simulink library "NxtrLim"  (R2013b)
settings: Solver=ode45  StartTime=0.0  StopTime=10.0  RelTol=1e-3
libraries: NxtrLim x2
settings Model: Creator=qzwc4r  LastModifiedBy=qzwc4r

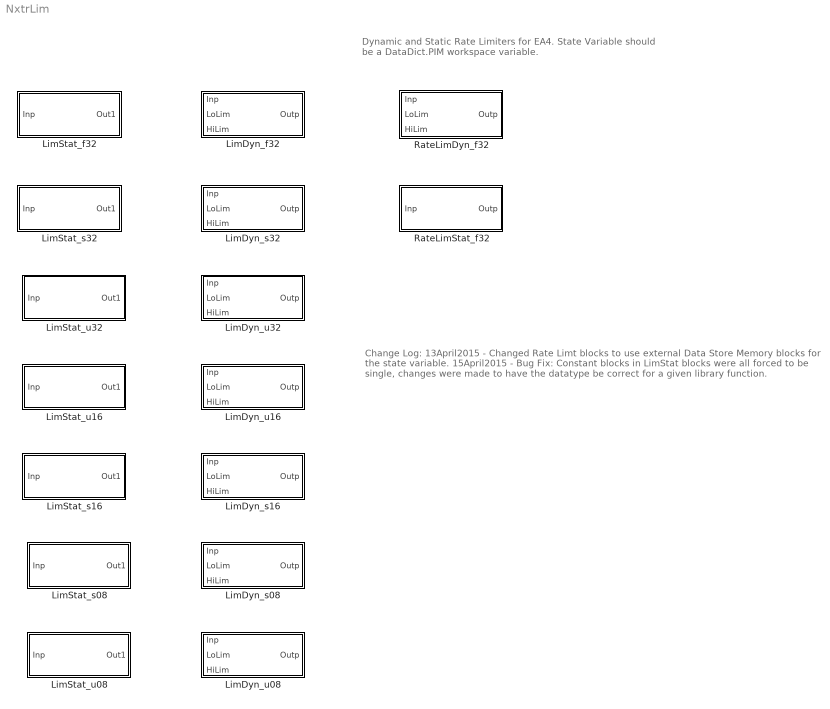
== system NxtrLim ==
  note: Change Log:
      |
      | 13April2015
      | - Changed Rate Limt blocks to use external Data Store Memory blocks for the state variable.
      |
      | 15April2015
      | - Bug Fix: Constant blocks in LimStat blocks were all forced to be single, changes were made
      |    to have the datatype be correct for a given library function.
  note: Dynamic and Static Rate Limiters for EA4.
      | State Variable should be a DataDict.PIM workspace variable.
  LimDyn_f32 : Subsystem  mask(LimDyn_f32){}
      mask Display:
      | Xx = [-0.06, 0.06]*3;
      | Xy = [ 0, 0];
      | Yx = [ 0, 0];
      | Yy = [-0.14, 0.14]*3;
      | 
      | px = [-.06, -0.02, 0.02, 0.06]*3;
      | py = [-.1, -.1, .1, .1]*3;
      | plot(Xx+.5,Xy+.5, Yx+.5,Yy+.5, px+.5,py+.5)
      | 
      | port_label('input',1,'Inp')
      | port_label('input',2,'LoLim')
      | port_label('input',3,'HiLim')
      | port_label('output',1,'Outp')
  LimDyn_s08 : Subsystem  mask(LimDyn_s08){}
      mask Display:
      | Xx = [-0.06, 0.06]*3;
      | Xy = [ 0, 0];
      | Yx = [ 0, 0];
      | Yy = [-0.14, 0.14]*3;
      | 
      | px = [-.06, -0.02, 0.02, 0.06]*3;
      | py = [-.1, -.1, .1, .1]*3;
      | plot(Xx+.5,Xy+.5, Yx+.5,Yy+.5, px+.5,py+.5)
      | 
      | port_label('input',1,'Inp')
      | port_label('input',2,'LoLim')
      | port_label('input',3,'HiLim')
      | port_label('output',1,'Outp')
  LimDyn_s16 : Subsystem  mask(LimDyn_s16){}
      mask Display:
      | Xx = [-0.06, 0.06]*3;
      | Xy = [ 0, 0];
      | Yx = [ 0, 0];
      | Yy = [-0.14, 0.14]*3;
      | 
      | px = [-.06, -0.02, 0.02, 0.06]*3;
      | py = [-.1, -.1, .1, .1]*3;
      | plot(Xx+.5,Xy+.5, Yx+.5,Yy+.5, px+.5,py+.5)
      | 
      | port_label('input',1,'Inp')
      | port_label('input',2,'LoLim')
      | port_label('input',3,'HiLim')
      | port_label('output',1,'Outp')
  LimDyn_s32 : Subsystem  mask(LimDyn_s32){}
      mask Display:
      | Xx = [-0.06, 0.06]*3;
      | Xy = [ 0, 0];
      | Yx = [ 0, 0];
      | Yy = [-0.14, 0.14]*3;
      | 
      | px = [-.06, -0.02, 0.02, 0.06]*3;
      | py = [-.1, -.1, .1, .1]*3;
      | plot(Xx+.5,Xy+.5, Yx+.5,Yy+.5, px+.5,py+.5)
      | 
      | port_label('input',1,'Inp')
      | port_label('input',2,'LoLim')
      | port_label('input',3,'HiLim')
      | port_label('output',1,'Outp')
  LimDyn_u08 : Subsystem  mask(LimDyn_u08){}
      mask Display:
      | Xx = [-0.06, 0.06]*3;
      | Xy = [ 0, 0];
      | Yx = [ 0, 0];
      | Yy = [-0.14, 0.14]*3;
      | 
      | px = [-.06, -0.02, 0.02, 0.06]*3;
      | py = [-.1, -.1, .1, .1]*3;
      | plot(Xx+.5,Xy+.5, Yx+.5,Yy+.5, px+.5,py+.5)
      | 
      | port_label('input',1,'Inp')
      | port_label('input',2,'LoLim')
      | port_label('input',3,'HiLim')
      | port_label('output',1,'Outp')
  LimDyn_u16 : Subsystem  mask(LimDyn_u16){}
      mask Display:
      | Xx = [-0.06, 0.06]*3;
      | Xy = [ 0, 0];
      | Yx = [ 0, 0];
      | Yy = [-0.14, 0.14]*3;
      | 
      | px = [-.06, -0.02, 0.02, 0.06]*3;
      | py = [-.1, -.1, .1, .1]*3;
      | plot(Xx+.5,Xy+.5, Yx+.5,Yy+.5, px+.5,py+.5)
      | 
      | port_label('input',1,'Inp')
      | port_label('input',2,'LoLim')
      | port_label('input',3,'HiLim')
      | port_label('output',1,'Outp')
  LimDyn_u32 : Subsystem  mask(LimDyn_u32){}
      mask Display:
      | Xx = [-0.06, 0.06]*3;
      | Xy = [ 0, 0];
      | Yx = [ 0, 0];
      | Yy = [-0.14, 0.14]*3;
      | 
      | px = [-.06, -0.02, 0.02, 0.06]*3;
      | py = [-.1, -.1, .1, .1]*3;
      | plot(Xx+.5,Xy+.5, Yx+.5,Yy+.5, px+.5,py+.5)
      | 
      | port_label('input',1,'Inp')
      | port_label('input',2,'LoLim')
      | port_label('input',3,'HiLim')
      | port_label('output',1,'Outp')
  LimStat_f32 : Subsystem  mask(LimStat_f32){LoLim=0, HiLim=0}
      mask prompts: LoLim "Lower Limit"; HiLim "Upper Limit"
      settings: AttributesFormatString=|
      | Low Limit: %<LoLim>
      | High Limit:%<HiLim>
      mask Display:
      | Xx = [-0.06, 0.06]*3;
      | Xy = [ 0, 0];
      | Yx = [ 0, 0];
      | Yy = [-0.14, 0.14]*3;
      | 
      | px = [-.06, -0.02, 0.02, 0.06]*3;
      | py = [-.1, -.1, .1, .1]*3;
      | plot(Xx+.5,Xy+.5, Yx+.5,Yy+.5, px+.5,py+.5)
      | 
      | port_label('input',1,'Inp')
      | port_label('output',1,'Outp')
  LimStat_s08 : Subsystem  mask(LimStat_s08){LoLim=0, HiLim=0}
      mask prompts: LoLim "Lower Limit"; HiLim "Upper Limit"
      settings: AttributesFormatString=|
      | Low Limit: %<LoLim>
      | High Limit:%<HiLim>
      mask Display:
      | Xx = [-0.06, 0.06]*3;
      | Xy = [ 0, 0];
      | Yx = [ 0, 0];
      | Yy = [-0.14, 0.14]*3;
      | 
      | px = [-.06, -0.02, 0.02, 0.06]*3;
      | py = [-.1, -.1, .1, .1]*3;
      | plot(Xx+.5,Xy+.5, Yx+.5,Yy+.5, px+.5,py+.5)
      | 
      | port_label('input',1,'Inp')
      | port_label('output',1,'Outp')
  LimStat_s16 : Subsystem  mask(LimStat_s16){LoLim=0, HiLim=0}
      mask prompts: LoLim "Lower Limit"; HiLim "Upper Limit"
      settings: AttributesFormatString=|
      | Low Limit: %<LoLim>
      | High Limit:%<HiLim>
      mask Display:
      | Xx = [-0.06, 0.06]*3;
      | Xy = [ 0, 0];
      | Yx = [ 0, 0];
      | Yy = [-0.14, 0.14]*3;
      | 
      | px = [-.06, -0.02, 0.02, 0.06]*3;
      | py = [-.1, -.1, .1, .1]*3;
      | plot(Xx+.5,Xy+.5, Yx+.5,Yy+.5, px+.5,py+.5)
      | 
      | port_label('input',1,'Inp')
      | port_label('output',1,'Outp')
  LimStat_s32 : Subsystem  mask(LimStat_s32){LoLim=0, HiLim=0}
      mask prompts: LoLim "Lower Limit"; HiLim "Upper Limit"
      settings: AttributesFormatString=|
      | Low Limit: %<LoLim>
      | High Limit:%<HiLim>
      mask Display:
      | Xx = [-0.06, 0.06]*3;
      | Xy = [ 0, 0];
      | Yx = [ 0, 0];
      | Yy = [-0.14, 0.14]*3;
      | 
      | px = [-.06, -0.02, 0.02, 0.06]*3;
      | py = [-.1, -.1, .1, .1]*3;
      | plot(Xx+.5,Xy+.5, Yx+.5,Yy+.5, px+.5,py+.5)
      | 
      | port_label('input',1,'Inp')
      | port_label('output',1,'Outp')
  LimStat_u08 : Subsystem  mask(LimStat_u08){LoLim=0, HiLim=0}
      mask prompts: LoLim "Lower Limit"; HiLim "Upper Limit"
      settings: AttributesFormatString=|
      | Low Limit: %<LoLim>
      | High Limit:%<HiLim>
      mask Display:
      | Xx = [-0.06, 0.06]*3;
      | Xy = [ 0, 0];
      | Yx = [ 0, 0];
      | Yy = [-0.14, 0.14]*3;
      | 
      | px = [-.06, -0.02, 0.02, 0.06]*3;
      | py = [-.1, -.1, .1, .1]*3;
      | plot(Xx+.5,Xy+.5, Yx+.5,Yy+.5, px+.5,py+.5)
      | 
      | port_label('input',1,'Inp')
      | port_label('output',1,'Outp')
  LimStat_u16 : Subsystem  mask(LimStat_u16){LoLim=0, HiLim=0}
      mask prompts: LoLim "Lower Limit"; HiLim "Upper Limit"
      settings: AttributesFormatString=|
      | Low Limit: %<LoLim>
      | High Limit:%<HiLim>
      mask Display:
      | Xx = [-0.06, 0.06]*3;
      | Xy = [ 0, 0];
      | Yx = [ 0, 0];
      | Yy = [-0.14, 0.14]*3;
      | 
      | px = [-.06, -0.02, 0.02, 0.06]*3;
      | py = [-.1, -.1, .1, .1]*3;
      | plot(Xx+.5,Xy+.5, Yx+.5,Yy+.5, px+.5,py+.5)
      | 
      | port_label('input',1,'Inp')
      | port_label('output',1,'Outp')
  LimStat_u32 : Subsystem  mask(LimStat_u32){LoLim=0, HiLim=0}
      mask prompts: LoLim "Lower Limit"; HiLim "Upper Limit"
      settings: AttributesFormatString=|
      | Low Limit: %<LoLim>
      | High Limit:%<HiLim>
      mask Display:
      | Xx = [-0.06, 0.06]*3;
      | Xy = [ 0, 0];
      | Yx = [ 0, 0];
      | Yy = [-0.14, 0.14]*3;
      | 
      | px = [-.06, -0.02, 0.02, 0.06]*3;
      | py = [-.1, -.1, .1, .1]*3;
      | plot(Xx+.5,Xy+.5, Yx+.5,Yy+.5, px+.5,py+.5)
      | 
      | port_label('input',1,'Inp')
      | port_label('output',1,'Outp')
  RateLimDyn_f32 : Subsystem  mask(RateLimDyn_f32){StVar=DefaultValue, Ts=0.002}
      mask prompts: StVar "State Variable"; Ts "Time Step"
      mask init:
      | blk = gcb;
      | set_param([ blk '/Data Store Write'],'DataStoreName',StVar)
      | set_param([ blk '/Data Store Read'],'DataStoreName',StVar)
      settings: AttributesFormatString=StVar: %<StVar>
      mask Display:
      | Xx = [-0.06, 0.06]*3;
      | Xy = [ 0, 0];
      | Yx = [ 0, 0];
      | Yy = [-0.14, 0.14]*3;
      | 
      | px = [-.15, 0.15];
      | py = [-.4, 0.4];
      | plot(Xx+.5,Xy+.5, Yx+.5,Yy+.5, px+.5,py+.5)
      | 
      | port_label('input',1,'Inp')
      | port_label('input',2,'LoLim')
      | port_label('input',3,'HiLim')
      | port_label('output',1,'Outp')
  RateLimStat_f32 : Subsystem  mask(RateLimStat_f32){StVar=DefaultValue, Ts=0.002, LoLim=0, HiLim=0}
      mask prompts: StVar "State Variable"; Ts "Time Step"; LoLim "Lower Limit"; HiLim "Upper Limit"
      mask init:
      | blk = gcb;
      | set_param([ blk '/Data Store Write'],'DataStoreName',StVar)
      | set_param([ blk '/Data Store Read'],'DataStoreName',StVar)
      settings: AttributesFormatString=|
      | StVar: %<StVar>
      | LoLim: %<LoLim>
      | HiLim: %<HiLim>
      mask Display:
      | Xx = [-0.06, 0.06]*3;
      | Xy = [ 0, 0];
      | Yx = [ 0, 0];
      | Yy = [-0.14, 0.14]*3;
      | 
      | px = [-.15, 0.15];
      | py = [-.4, 0.4];
      | plot(Xx+.5,Xy+.5, Yx+.5,Yy+.5, px+.5,py+.5)
      | 
      | port_label('input',1,'Inp')
      | port_label('output',1,'Outp')

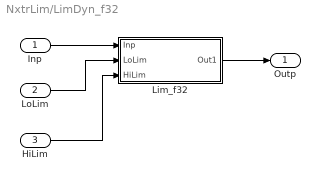
== system NxtrLim/LimDyn_f32 ==
  Inp : Inport
  LoLim : Inport  Port=2
  HiLim : Inport  Port=3
  Lim_f32 : Subsystem
      mask Display:
      | port_label('input',1,'Inp')
      | port_label('input',2,'LoLim')
      | port_label('input',3,'HiLim')
      | port_label('output',1,'Outp')
  Outp : Outport
  wires:
  Lim_f32/1(Out1) -> Outp/1
  Inp/1 -> Lim_f32/1(Inp)
  LoLim/1 -> Lim_f32/2(LoLim)
  HiLim/1 -> Lim_f32/3(HiLim)

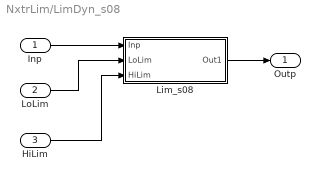
== system NxtrLim/LimDyn_s08 ==
  Inp : Inport
  LoLim : Inport  Port=2
  HiLim : Inport  Port=3
  Lim_s08 : Subsystem
      mask Display:
      | Xx = [-0.06, 0.06]*3;
      | Xy = [ 0, 0];
      | Yx = [ 0, 0];
      | Yy = [-0.14, 0.14]*3;
      | 
      | px = [-.06, -0.02, 0.02, 0.06]*3;
      | py = [-.1, -.1, .1, .1]*3;
      | plot(Xx+.5,Xy+.5, Yx+.5,Yy+.5, px+.5,py+.5)
      | 
      | port_label('input',1,'Inp')
      | port_label('input',2,'LoLim')
      | port_label('input',3,'HiLim')
      | port_label('output',1,'Outp')
  Outp : Outport
  wires:
  HiLim/1 -> Lim_s08/3(HiLim)
  LoLim/1 -> Lim_s08/2(LoLim)
  Inp/1 -> Lim_s08/1(Inp)
  Lim_s08/1(Out1) -> Outp/1

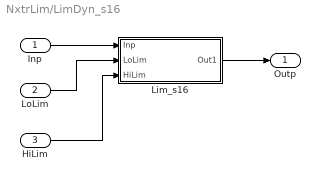
== system NxtrLim/LimDyn_s16 ==
  Inp : Inport
  LoLim : Inport  Port=2
  HiLim : Inport  Port=3
  Lim_s16 : Subsystem
      mask Display:
      | Xx = [-0.06, 0.06]*3;
      | Xy = [ 0, 0];
      | Yx = [ 0, 0];
      | Yy = [-0.14, 0.14]*3;
      | 
      | px = [-.06, -0.02, 0.02, 0.06]*3;
      | py = [-.1, -.1, .1, .1]*3;
      | plot(Xx+.5,Xy+.5, Yx+.5,Yy+.5, px+.5,py+.5)
      | 
      | port_label('input',1,'Inp')
      | port_label('input',2,'LoLim')
      | port_label('input',3,'HiLim')
      | port_label('output',1,'Outp')
  Outp : Outport
  wires:
  Lim_s16/1(Out1) -> Outp/1
  Inp/1 -> Lim_s16/1(Inp)
  LoLim/1 -> Lim_s16/2(LoLim)
  HiLim/1 -> Lim_s16/3(HiLim)

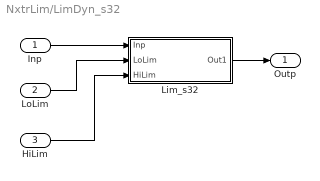
== system NxtrLim/LimDyn_s32 ==
  Inp : Inport
  LoLim : Inport  Port=2
  HiLim : Inport  Port=3
  Lim_s32 : Subsystem
      mask Display:
      | Xx = [-0.06, 0.06]*3;
      | Xy = [ 0, 0];
      | Yx = [ 0, 0];
      | Yy = [-0.14, 0.14]*3;
      | 
      | px = [-.06, -0.02, 0.02, 0.06]*3;
      | py = [-.1, -.1, .1, .1]*3;
      | plot(Xx+.5,Xy+.5, Yx+.5,Yy+.5, px+.5,py+.5)
      | 
      | port_label('input',1,'Inp')
      | port_label('input',2,'LoLim')
      | port_label('input',3,'HiLim')
      | port_label('output',1,'Outp')
  Outp : Outport
  wires:
  HiLim/1 -> Lim_s32/3(HiLim)
  LoLim/1 -> Lim_s32/2(LoLim)
  Inp/1 -> Lim_s32/1(Inp)
  Lim_s32/1(Out1) -> Outp/1

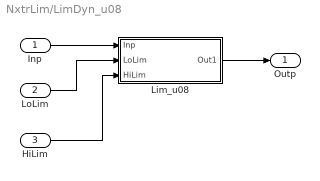
== system NxtrLim/LimDyn_u08 ==
  Inp : Inport
  LoLim : Inport  Port=2
  HiLim : Inport  Port=3
  Lim_u08 : Subsystem
      mask Display:
      | Xx = [-0.06, 0.06]*3;
      | Xy = [ 0, 0];
      | Yx = [ 0, 0];
      | Yy = [-0.14, 0.14]*3;
      | 
      | px = [-.06, -0.02, 0.02, 0.06]*3;
      | py = [-.1, -.1, .1, .1]*3;
      | plot(Xx+.5,Xy+.5, Yx+.5,Yy+.5, px+.5,py+.5)
      | 
      | port_label('input',1,'Inp')
      | port_label('input',2,'LoLim')
      | port_label('input',3,'HiLim')
      | port_label('output',1,'Outp')
  Outp : Outport
  wires:
  Lim_u08/1(Out1) -> Outp/1
  Inp/1 -> Lim_u08/1(Inp)
  LoLim/1 -> Lim_u08/2(LoLim)
  HiLim/1 -> Lim_u08/3(HiLim)

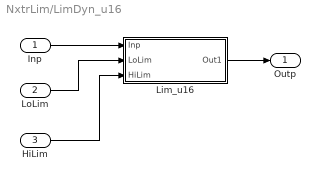
== system NxtrLim/LimDyn_u16 ==
  Inp : Inport
  LoLim : Inport  Port=2
  HiLim : Inport  Port=3
  Lim_u16 : Subsystem
      mask Display:
      | Xx = [-0.06, 0.06]*3;
      | Xy = [ 0, 0];
      | Yx = [ 0, 0];
      | Yy = [-0.14, 0.14]*3;
      | 
      | px = [-.06, -0.02, 0.02, 0.06]*3;
      | py = [-.1, -.1, .1, .1]*3;
      | plot(Xx+.5,Xy+.5, Yx+.5,Yy+.5, px+.5,py+.5)
      | 
      | port_label('input',1,'Inp')
      | port_label('input',2,'LoLim')
      | port_label('input',3,'HiLim')
      | port_label('output',1,'Outp')
  Outp : Outport
  wires:
  HiLim/1 -> Lim_u16/3(HiLim)
  LoLim/1 -> Lim_u16/2(LoLim)
  Inp/1 -> Lim_u16/1(Inp)
  Lim_u16/1(Out1) -> Outp/1

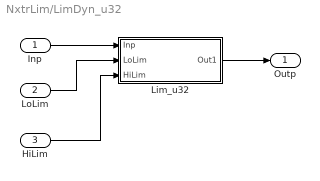
== system NxtrLim/LimDyn_u32 ==
  Inp : Inport
  LoLim : Inport  Port=2
  HiLim : Inport  Port=3
  Lim_u32 : Subsystem
      mask Display:
      | Xx = [-0.06, 0.06]*3;
      | Xy = [ 0, 0];
      | Yx = [ 0, 0];
      | Yy = [-0.14, 0.14]*3;
      | 
      | px = [-.06, -0.02, 0.02, 0.06]*3;
      | py = [-.1, -.1, .1, .1]*3;
      | plot(Xx+.5,Xy+.5, Yx+.5,Yy+.5, px+.5,py+.5)
      | 
      | port_label('input',1,'Inp')
      | port_label('input',2,'LoLim')
      | port_label('input',3,'HiLim')
      | port_label('output',1,'Outp')
  Outp : Outport
  wires:
  Lim_u32/1(Out1) -> Outp/1
  Inp/1 -> Lim_u32/1(Inp)
  LoLim/1 -> Lim_u32/2(LoLim)
  HiLim/1 -> Lim_u32/3(HiLim)

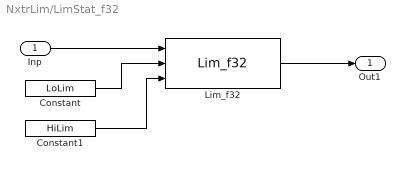
== system NxtrLim/LimStat_f32 ==
  Inp : Inport
  Constant : Constant  Value=LoLim  OutDataTypeStr=single
  Constant1 : Constant  Value=HiLim  OutDataTypeStr=single
  Lim_f32 : S-Function  FunctionName=Lim_f32  EnableBusSupport=off  mask(Legacy Function){SFunctionSpec=single y1 = Lim_f32(single u1, single u2, single u3)}
      mask help:
      | This block allows you to call the legacy functions specified by the following Legacy Code Tool definition:
      | def.SFunctionName = 'Lim_f32';
      | def.OutputFcnSpec = 'single y1 = Lim_f32(single u1, single u2, single u3)';
      | def.HeaderFiles = {'NxtrMath.h', 'Std_Types.h', 'Platform_Types.h', 'Compiler.h', 'Compiler_Cfg.h'};
      | def.IncPaths = {'..\Nexteer_Utilities v3.0.0\SrcFiles'};
      settings: AttributesFormatString=%<Name>
      mask Help: <p>This block was generated automatically by the Legacy Code Tool. For detailed help on this tool, call<a href="matlab:legacy_code('help')"> legacy_code('help')</a>.</p>
      mask Display:
      | port_label('input',1,'Inp')
      | port_label('input',2,'LoLim')
      | port_label('input',3,'HiLim')
      | port_label('output',1,'Outp')
  Out1 : Outport
  wires:
  Lim_f32/1 -> Out1/1
  Constant1/1 -> Lim_f32/3
  Constant/1 -> Lim_f32/2
  Inp/1 -> Lim_f32/1

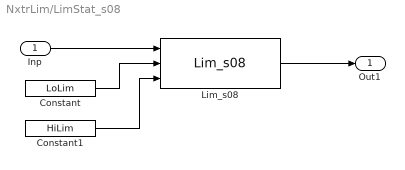
== system NxtrLim/LimStat_s08 ==
  Inp : Inport
  Constant : Constant  Value=LoLim  OutDataTypeStr=int8
  Constant1 : Constant  Value=HiLim  OutDataTypeStr=int8
  Lim_s08 : S-Function  FunctionName=Lim_s08  EnableBusSupport=off  mask(Legacy Function){SFunctionSpec=int8 y1 = Lim_s08(  int8 u1,   int8 u2,   int8 u3), ShowSpec=on}
      mask prompts: ShowSpec "Display function specification"
      mask help:
      | This block allows you to call the legacy functions specified by the following Legacy Code Tool definition:
      | def.SFunctionName = 'Lim_s08';
      | def.OutputFcnSpec = '  int8 y1 = Lim_s08(  int8 u1,   int8 u2,   int8 u3)';
      | def.HeaderFiles = {'NxtrMath.h', 'Std_Types.h', 'Platform_Types.h', 'Compiler.h', 'Compiler_Cfg.h'};
      | def.IncPaths = {'..\Nexteer_Utilities v3.0.0\SrcFiles'};
      settings: AttributesFormatString=%<Name>
      mask Help: <p>This block was generated automatically by the Legacy Code Tool. For detailed help on this tool, call<a href="matlab:legacy_code('help')"> legacy_code('help')</a>.</p>
      mask Callback ShowSpec:
      | if strcmp(get_param(gcbh, 'ShowSpec'), 'on')
      |   set_param(gcbh, 'MaskDisplay', sprintf('fprintf(''%s'');', get_param(gcbh, 'SFunctionSpec')));
      | else
      |   set_param(gcbh, 'MaskDisplay', sprintf('fprintf(''%s'');', get_param(gcbh, 'FunctionName')));
      | end
      mask Display:
      | Xx = [-0.06, 0.06]*3;
      | Xy = [ 0, 0];
      | Yx = [ 0, 0];
      | Yy = [-0.14, 0.14]*3;
      | 
      | px = [-.06, -0.02, 0.02, 0.06]*3;
      | py = [-.1, -.1, .1, .1]*3;
      | plot(Xx+.5,Xy+.5, Yx+.5,Yy+.5, px+.5,py+.5)
      | port_label('input',1,'Inp')
      | port_label('input',2,'LoLim')
      | port_label('input',3,'HiLim')
      | port_label('output',1,'Outp')
  Out1 : Outport
  wires:
  Inp/1 -> Lim_s08/1
  Constant/1 -> Lim_s08/2
  Constant1/1 -> Lim_s08/3
  Lim_s08/1 -> Out1/1

== system NxtrLim/LimStat_s16 ==
  Inp : Inport
  Constant : Constant  Value=LoLim  OutDataTypeStr=int16
  Constant1 : Constant  Value=HiLim  OutDataTypeStr=int16
  Lim_s16 : S-Function  FunctionName=Lim_s16  EnableBusSupport=off  mask(Legacy Function){SFunctionSpec=int16 y1 = Lim_s16( int16 u1,  int16 u2,  int16 u3)}
      mask help:
      | This block allows you to call the legacy functions specified by the following Legacy Code Tool definition:
      | def.SFunctionName = 'Lim_s16';
      | def.OutputFcnSpec = ' int16 y1 = Lim_s16( int16 u1,  int16 u2,  int16 u3)';
      | def.HeaderFiles = {'NxtrMath.h', 'Std_Types.h', 'Platform_Types.h', 'Compiler.h', 'Compiler_Cfg.h'};
      | def.IncPaths = {'..\Nexteer_Utilities v3.0.0\SrcFiles'};
      settings: AttributesFormatString=%<Name>
      mask Help: <p>This block was generated automatically by the Legacy Code Tool. For detailed help on this tool, call<a href="matlab:legacy_code('help')"> legacy_code('help')</a>.</p>
      mask Display:
      | Xx = [-0.06, 0.06]*3;
      | Xy = [ 0, 0];
      | Yx = [ 0, 0];
      | Yy = [-0.14, 0.14]*3;
      | 
      | px = [-.06, -0.02, 0.02, 0.06]*3;
      | py = [-.1, -.1, .1, .1]*3;
      | plot(Xx+.5,Xy+.5, Yx+.5,Yy+.5, px+.5,py+.5)
      | port_label('input',1,'Inp')
      | port_label('input',2,'LoLim')
      | port_label('input',3,'HiLim')
      | port_label('output',1,'Outp')
  Out1 : Outport
  wires:
  Lim_s16/1 -> Out1/1
  Constant1/1 -> Lim_s16/3
  Constant/1 -> Lim_s16/2
  Inp/1 -> Lim_s16/1

== system NxtrLim/LimStat_s32 ==
  Inp : Inport
  Constant : Constant  Value=LoLim  OutDataTypeStr=int32
  Constant1 : Constant  Value=HiLim  OutDataTypeStr=int32
  Lim_s32 : Subsystem
      mask Display:
      | Xx = [-0.06, 0.06]*3;
      | Xy = [ 0, 0];
      | Yx = [ 0, 0];
      | Yy = [-0.14, 0.14]*3;
      | 
      | px = [-.06, -0.02, 0.02, 0.06]*3;
      | py = [-.1, -.1, .1, .1]*3;
      | plot(Xx+.5,Xy+.5, Yx+.5,Yy+.5, px+.5,py+.5)
      | 
      | port_label('input',1,'Inp')
      | port_label('input',2,'LoLim')
      | port_label('input',3,'HiLim')
      | port_label('output',1,'Outp')
  Out1 : Outport
  wires:
  Inp/1 -> Lim_s32/1(Inp)
  Constant/1 -> Lim_s32/2(LoLim)
  Constant1/1 -> Lim_s32/3(HiLim)
  Lim_s32/1(Out1) -> Out1/1

== system NxtrLim/LimStat_u08 ==
  Inp : Inport
  Constant : Constant  Value=LoLim  OutDataTypeStr=uint8
  Constant1 : Constant  Value=HiLim  OutDataTypeStr=uint8
  Lim_u08 : S-Function  FunctionName=Lim_u08  EnableBusSupport=off  mask(Legacy Function){SFunctionSpec=uint8 y1 = Lim_u08( uint8 u1,  uint8 u2,  uint8 u3), ShowSpec=on}
      mask prompts: ShowSpec "Display function specification"
      mask help:
      | This block allows you to call the legacy functions specified by the following Legacy Code Tool definition:
      | def.SFunctionName = 'Lim_u08';
      | def.OutputFcnSpec = ' uint8 y1 = Lim_u08( uint8 u1,  uint8 u2,  uint8 u3)';
      | def.HeaderFiles = {'NxtrMath.h', 'Std_Types.h', 'Platform_Types.h', 'Compiler.h', 'Compiler_Cfg.h'};
      | def.IncPaths = {'..\Nexteer_Utilities v3.0.0\SrcFiles'};
      settings: AttributesFormatString=%<Name>
      mask Help: <p>This block was generated automatically by the Legacy Code Tool. For detailed help on this tool, call<a href="matlab:legacy_code('help')"> legacy_code('help')</a>.</p>
      mask Callback ShowSpec:
      | if strcmp(get_param(gcbh, 'ShowSpec'), 'on')
      |   set_param(gcbh, 'MaskDisplay', sprintf('fprintf(''%s'');', get_param(gcbh, 'SFunctionSpec')));
      | else
      |   set_param(gcbh, 'MaskDisplay', sprintf('fprintf(''%s'');', get_param(gcbh, 'FunctionName')));
      | end
      mask Display:
      | Xx = [-0.06, 0.06]*3;
      | Xy = [ 0, 0];
      | Yx = [ 0, 0];
      | Yy = [-0.14, 0.14]*3;
      | 
      | px = [-.06, -0.02, 0.02, 0.06]*3;
      | py = [-.1, -.1, .1, .1]*3;
      | plot(Xx+.5,Xy+.5, Yx+.5,Yy+.5, px+.5,py+.5)
      | port_label('input',1,'Inp')
      | port_label('input',2,'LoLim')
      | port_label('input',3,'HiLim')
      | port_label('output',1,'Outp')
  Out1 : Outport
  wires:
  Lim_u08/1 -> Out1/1
  Constant1/1 -> Lim_u08/3
  Constant/1 -> Lim_u08/2
  Inp/1 -> Lim_u08/1

== system NxtrLim/LimStat_u16 ==
  Inp : Inport
  Constant : Constant  Value=LoLim  OutDataTypeStr=uint16
  Constant1 : Constant  Value=HiLim  OutDataTypeStr=uint16
  Lim_u16 : S-Function  FunctionName=Lim_u16  EnableBusSupport=off  mask(Legacy Function){SFunctionSpec=uint16 y1 = Lim_u16(uint16 u1, uint16 u2, uint16 u3)}
      mask help:
      | This block allows you to call the legacy functions specified by the following Legacy Code Tool definition:
      | def.SFunctionName = 'Lim_u16';
      | def.OutputFcnSpec = 'uint16 y1 = Lim_u16(uint16 u1, uint16 u2, uint16 u3)';
      | def.HeaderFiles = {'NxtrMath.h', 'Std_Types.h', 'Platform_Types.h', 'Compiler.h', 'Compiler_Cfg.h'};
      | def.IncPaths = {'..\Nexteer_Utilities v3.0.0\SrcFiles'};
      settings: AttributesFormatString=%<Name>
      mask Help: <p>This block was generated automatically by the Legacy Code Tool. For detailed help on this tool, call<a href="matlab:legacy_code('help')"> legacy_code('help')</a>.</p>
      mask Display:
      | Xx = [-0.06, 0.06]*3;
      | Xy = [ 0, 0];
      | Yx = [ 0, 0];
      | Yy = [-0.14, 0.14]*3;
      | 
      | px = [-.06, -0.02, 0.02, 0.06]*3;
      | py = [-.1, -.1, .1, .1]*3;
      | plot(Xx+.5,Xy+.5, Yx+.5,Yy+.5, px+.5,py+.5)
      | port_label('input',1,'Inp')
      | port_label('input',2,'LoLim')
      | port_label('input',3,'HiLim')
      | port_label('output',1,'Outp')
  Out1 : Outport
  wires:
  Inp/1 -> Lim_u16/1
  Constant/1 -> Lim_u16/2
  Constant1/1 -> Lim_u16/3
  Lim_u16/1 -> Out1/1

== system NxtrLim/LimStat_u32 ==
  Inp : Inport
  Constant : Constant  Value=LoLim  OutDataTypeStr=uint32
  Constant1 : Constant  Value=HiLim  OutDataTypeStr=uint32
  Lim_u32 : S-Function  FunctionName=Lim_u32  EnableBusSupport=off  mask(Legacy Function){SFunctionSpec=uint32 y1 = Lim_u32(uint32 u1, uint32 u2, uint32 u3)}
      mask help:
      | This block allows you to call the legacy functions specified by the following Legacy Code Tool definition:
      | def.SFunctionName = 'Lim_u32';
      | def.OutputFcnSpec = 'uint32 y1 = Lim_u32(uint32 u1, uint32 u2, uint32 u3)';
      | def.HeaderFiles = {'NxtrMath.h', 'Std_Types.h', 'Platform_Types.h', 'Compiler.h', 'Compiler_Cfg.h'};
      | def.IncPaths = {'..\Nexteer_Utilities v3.0.0\SrcFiles'};
      settings: AttributesFormatString=%<Name>
      mask Help: <p>This block was generated automatically by the Legacy Code Tool. For detailed help on this tool, call<a href="matlab:legacy_code('help')"> legacy_code('help')</a>.</p>
      mask Display:
      | Xx = [-0.06, 0.06]*3;
      | Xy = [ 0, 0];
      | Yx = [ 0, 0];
      | Yy = [-0.14, 0.14]*3;
      | 
      | px = [-.06, -0.02, 0.02, 0.06]*3;
      | py = [-.1, -.1, .1, .1]*3;
      | plot(Xx+.5,Xy+.5, Yx+.5,Yy+.5, px+.5,py+.5)
      | port_label('input',1,'Inp')
      | port_label('input',2,'LoLim')
      | port_label('input',3,'HiLim')
      | port_label('output',1,'Outp')
  Out1 : Outport
  wires:
  Lim_u32/1 -> Out1/1
  Constant1/1 -> Lim_u32/3
  Constant/1 -> Lim_u32/2
  Inp/1 -> Lim_u32/1

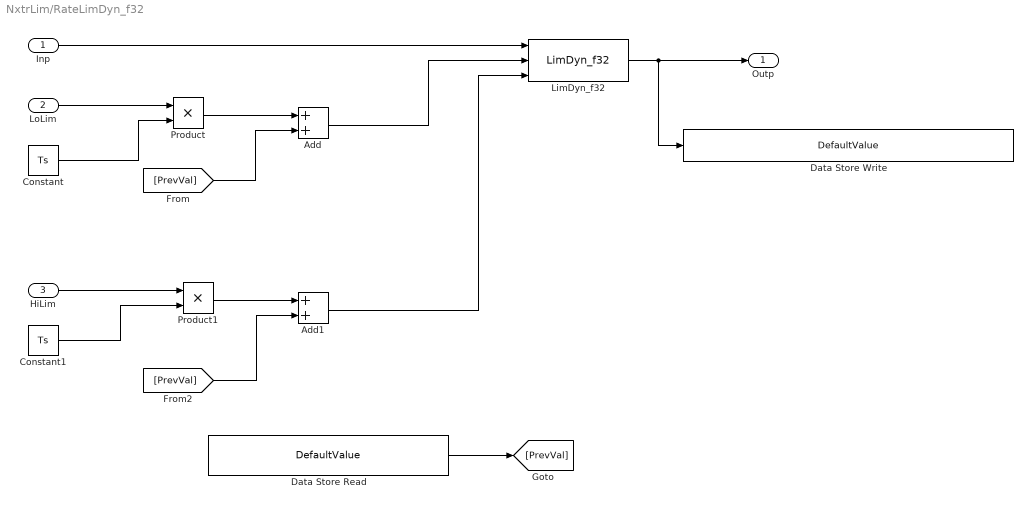
== system NxtrLim/RateLimDyn_f32 ==
  Inp : Inport
  LoLim : Inport  Port=2
  HiLim : Inport  Port=3
  Add : Sum
  Add1 : Sum
  Constant : Constant  Value=Ts
  Constant1 : Constant  Value=Ts
  Data Store Read : DataStoreRead  DataStoreName=DefaultValue
  Data Store Write : DataStoreWrite  DataStoreName=DefaultValue
  LimDyn_f32 : NxtrLim/LimDyn_f32
  Product : Product
  Product1 : Product
  Outp : Outport
  wires:
  Inp/1 -> LimDyn_f32/1
  LimDyn_f32/1 -> Data Store Write/1, Outp/1
  Data Store Read/1 -> [PrevVal]
  LoLim/1 -> Product/1
  Constant/1 -> Product/2
  Product/1 -> Add/1
  HiLim/1 -> Product1/1
  Constant1/1 -> Product1/2
  Product1/1 -> Add1/1
  Add/1 -> LimDyn_f32/2
  Add1/1 -> LimDyn_f32/3
  [PrevVal] -> Add/2
  [PrevVal] -> Add1/2

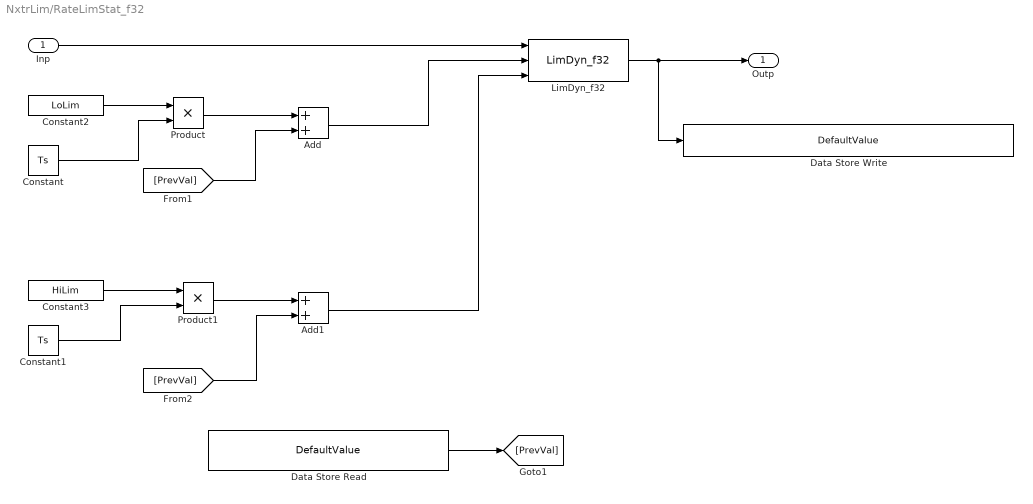
== system NxtrLim/RateLimStat_f32 ==
  Inp : Inport
  Add : Sum
  Add1 : Sum
  Constant : Constant  Value=Ts
  Constant1 : Constant  Value=Ts
  Constant2 : Constant  Value=LoLim
  Constant3 : Constant  Value=HiLim
  Data Store Read : DataStoreRead  DataStoreName=DefaultValue
  Data Store Write : DataStoreWrite  DataStoreName=DefaultValue
  LimDyn_f32 : NxtrLim/LimDyn_f32
  Product : Product
  Product1 : Product
  Outp : Outport
  wires:
  [PrevVal] -> Add1/2
  [PrevVal] -> Add/2
  Add1/1 -> LimDyn_f32/3
  Add/1 -> LimDyn_f32/2
  Product1/1 -> Add1/1
  Constant1/1 -> Product1/2
  Constant3/1 -> Product1/1
  Product/1 -> Add/1
  Constant/1 -> Product/2
  Constant2/1 -> Product/1
  Data Store Read/1 -> [PrevVal]
  LimDyn_f32/1 -> Data Store Write/1, Outp/1
  Inp/1 -> LimDyn_f32/1

== system NxtrLim/LimDyn_f32/Lim_f32 ==
  Inp : Inport
  LoLim : Inport  Port=2
  HiLim : Inport  Port=3
  Lim_f32 : S-Function  FunctionName=Lim_f32  EnableBusSupport=off  mask(Legacy Function){SFunctionSpec=single y1 = Lim_f32(single u1, single u2, single u3)}
      mask help:
      | This block allows you to call the legacy functions specified by the following Legacy Code Tool definition:
      | def.SFunctionName = 'Lim_f32';
      | def.OutputFcnSpec = 'single y1 = Lim_f32(single u1, single u2, single u3)';
      | def.HeaderFiles = {'NxtrMath.h', 'Std_Types.h', 'Platform_Types.h', 'Compiler.h', 'Compiler_Cfg.h'};
      | def.IncPaths = {'..\Nexteer_Utilities v3.0.0\SrcFiles'};
      settings: AttributesFormatString=%<Name>
      mask Help: <p>This block was generated automatically by the Legacy Code Tool. For detailed help on this tool, call<a href="matlab:legacy_code('help')"> legacy_code('help')</a>.</p>
      mask Display:
      | port_label('input',1,'Inp')
      | port_label('input',2,'LoLim')
      | port_label('input',3,'HiLim')
      | port_label('output',1,'Outp')
  Out1 : Outport
  wires:
  Lim_f32/1 -> Out1/1
  HiLim/1 -> Lim_f32/3
  LoLim/1 -> Lim_f32/2
  Inp/1 -> Lim_f32/1

== system NxtrLim/LimDyn_s08/Lim_s08 ==
  Inp : Inport
  LoLim : Inport  Port=2
  HiLim : Inport  Port=3
  Lim_s08 : S-Function  FunctionName=Lim_s08  EnableBusSupport=off  mask(Legacy Function){SFunctionSpec=int8 y1 = Lim_s08(  int8 u1,   int8 u2,   int8 u3), ShowSpec=on}
      mask prompts: ShowSpec "Display function specification"
      mask help:
      | This block allows you to call the legacy functions specified by the following Legacy Code Tool definition:
      | def.SFunctionName = 'Lim_s08';
      | def.OutputFcnSpec = '  int8 y1 = Lim_s08(  int8 u1,   int8 u2,   int8 u3)';
      | def.HeaderFiles = {'NxtrMath.h', 'Std_Types.h', 'Platform_Types.h', 'Compiler.h', 'Compiler_Cfg.h'};
      | def.IncPaths = {'..\Nexteer_Utilities v3.0.0\SrcFiles'};
      settings: AttributesFormatString=%<Name>
      mask Help: <p>This block was generated automatically by the Legacy Code Tool. For detailed help on this tool, call<a href="matlab:legacy_code('help')"> legacy_code('help')</a>.</p>
      mask Callback ShowSpec:
      | if strcmp(get_param(gcbh, 'ShowSpec'), 'on')
      |   set_param(gcbh, 'MaskDisplay', sprintf('fprintf(''%s'');', get_param(gcbh, 'SFunctionSpec')));
      | else
      |   set_param(gcbh, 'MaskDisplay', sprintf('fprintf(''%s'');', get_param(gcbh, 'FunctionName')));
      | end
      mask Display:
      | Xx = [-0.06, 0.06]*3;
      | Xy = [ 0, 0];
      | Yx = [ 0, 0];
      | Yy = [-0.14, 0.14]*3;
      | 
      | px = [-.06, -0.02, 0.02, 0.06]*3;
      | py = [-.1, -.1, .1, .1]*3;
      | plot(Xx+.5,Xy+.5, Yx+.5,Yy+.5, px+.5,py+.5)
      | port_label('input',1,'Inp')
      | port_label('input',2,'LoLim')
      | port_label('input',3,'HiLim')
      | port_label('output',1,'Outp')
  Out1 : Outport
  wires:
  Inp/1 -> Lim_s08/1
  LoLim/1 -> Lim_s08/2
  HiLim/1 -> Lim_s08/3
  Lim_s08/1 -> Out1/1

== system NxtrLim/LimDyn_s16/Lim_s16 ==
  Inp : Inport
  LoLim : Inport  Port=2
  HiLim : Inport  Port=3
  Lim_s16 : S-Function  FunctionName=Lim_s16  EnableBusSupport=off  mask(Legacy Function){SFunctionSpec=int16 y1 = Lim_s16( int16 u1,  int16 u2,  int16 u3)}
      mask help:
      | This block allows you to call the legacy functions specified by the following Legacy Code Tool definition:
      | def.SFunctionName = 'Lim_s16';
      | def.OutputFcnSpec = ' int16 y1 = Lim_s16( int16 u1,  int16 u2,  int16 u3)';
      | def.HeaderFiles = {'NxtrMath.h', 'Std_Types.h', 'Platform_Types.h', 'Compiler.h', 'Compiler_Cfg.h'};
      | def.IncPaths = {'..\Nexteer_Utilities v3.0.0\SrcFiles'};
      settings: AttributesFormatString=%<Name>
      mask Help: <p>This block was generated automatically by the Legacy Code Tool. For detailed help on this tool, call<a href="matlab:legacy_code('help')"> legacy_code('help')</a>.</p>
      mask Display:
      | Xx = [-0.06, 0.06]*3;
      | Xy = [ 0, 0];
      | Yx = [ 0, 0];
      | Yy = [-0.14, 0.14]*3;
      | 
      | px = [-.06, -0.02, 0.02, 0.06]*3;
      | py = [-.1, -.1, .1, .1]*3;
      | plot(Xx+.5,Xy+.5, Yx+.5,Yy+.5, px+.5,py+.5)
      | port_label('input',1,'Inp')
      | port_label('input',2,'LoLim')
      | port_label('input',3,'HiLim')
      | port_label('output',1,'Outp')
  Out1 : Outport
  wires:
  Lim_s16/1 -> Out1/1
  HiLim/1 -> Lim_s16/3
  LoLim/1 -> Lim_s16/2
  Inp/1 -> Lim_s16/1

== system NxtrLim/LimDyn_s32/Lim_s32 ==
  Inp : Inport
  LoLim : Inport  Port=2
  HiLim : Inport  Port=3
  Lim_s32 : S-Function  FunctionName=Lim_s32  EnableBusSupport=off  mask(Legacy Function){SFunctionSpec=int32 y1 = Lim_s32( int32 u1,  int32 u2,  int32 u3)}
      mask help:
      | This block allows you to call the legacy functions specified by the following Legacy Code Tool definition:
      | def.SFunctionName = 'Lim_s32';
      | def.OutputFcnSpec = ' int32 y1 = Lim_s32( int32 u1,  int32 u2,  int32 u3)';
      | def.HeaderFiles = {'NxtrMath.h', 'Std_Types.h', 'Platform_Types.h', 'Compiler.h', 'Compiler_Cfg.h'};
      | def.IncPaths = {'..\Nexteer_Utilities v3.0.0\SrcFiles'};
      settings: AttributesFormatString=%<Name>
      mask Help: <p>This block was generated automatically by the Legacy Code Tool. For detailed help on this tool, call<a href="matlab:legacy_code('help')"> legacy_code('help')</a>.</p>
      mask Display:
      | Xx = [-0.06, 0.06]*3;
      | Xy = [ 0, 0];
      | Yx = [ 0, 0];
      | Yy = [-0.14, 0.14]*3;
      | 
      | px = [-.06, -0.02, 0.02, 0.06]*3;
      | py = [-.1, -.1, .1, .1]*3;
      | plot(Xx+.5,Xy+.5, Yx+.5,Yy+.5, px+.5,py+.5)
      | port_label('input',1,'Inp')
      | port_label('input',2,'LoLim')
      | port_label('input',3,'HiLim')
      | port_label('output',1,'Outp')
  Out1 : Outport
  wires:
  Inp/1 -> Lim_s32/1
  LoLim/1 -> Lim_s32/2
  HiLim/1 -> Lim_s32/3
  Lim_s32/1 -> Out1/1

== system NxtrLim/LimDyn_u08/Lim_u08 ==
  Inp : Inport
  LoLim : Inport  Port=2
  HiLim : Inport  Port=3
  Lim_u08 : S-Function  FunctionName=Lim_u08  EnableBusSupport=off  mask(Legacy Function){SFunctionSpec=uint8 y1 = Lim_u08( uint8 u1,  uint8 u2,  uint8 u3), ShowSpec=on}
      mask prompts: ShowSpec "Display function specification"
      mask help:
      | This block allows you to call the legacy functions specified by the following Legacy Code Tool definition:
      | def.SFunctionName = 'Lim_u08';
      | def.OutputFcnSpec = ' uint8 y1 = Lim_u08( uint8 u1,  uint8 u2,  uint8 u3)';
      | def.HeaderFiles = {'NxtrMath.h', 'Std_Types.h', 'Platform_Types.h', 'Compiler.h', 'Compiler_Cfg.h'};
      | def.IncPaths = {'..\Nexteer_Utilities v3.0.0\SrcFiles'};
      settings: AttributesFormatString=%<Name>
      mask Help: <p>This block was generated automatically by the Legacy Code Tool. For detailed help on this tool, call<a href="matlab:legacy_code('help')"> legacy_code('help')</a>.</p>
      mask Callback ShowSpec:
      | if strcmp(get_param(gcbh, 'ShowSpec'), 'on')
      |   set_param(gcbh, 'MaskDisplay', sprintf('fprintf(''%s'');', get_param(gcbh, 'SFunctionSpec')));
      | else
      |   set_param(gcbh, 'MaskDisplay', sprintf('fprintf(''%s'');', get_param(gcbh, 'FunctionName')));
      | end
      mask Display:
      | Xx = [-0.06, 0.06]*3;
      | Xy = [ 0, 0];
      | Yx = [ 0, 0];
      | Yy = [-0.14, 0.14]*3;
      | 
      | px = [-.06, -0.02, 0.02, 0.06]*3;
      | py = [-.1, -.1, .1, .1]*3;
      | plot(Xx+.5,Xy+.5, Yx+.5,Yy+.5, px+.5,py+.5)
      | port_label('input',1,'Inp')
      | port_label('input',2,'LoLim')
      | port_label('input',3,'HiLim')
      | port_label('output',1,'Outp')
  Out1 : Outport
  wires:
  Lim_u08/1 -> Out1/1
  HiLim/1 -> Lim_u08/3
  LoLim/1 -> Lim_u08/2
  Inp/1 -> Lim_u08/1

== system NxtrLim/LimDyn_u16/Lim_u16 ==
  Inp : Inport
  LoLim : Inport  Port=2
  HiLim : Inport  Port=3
  Lim_u16 : S-Function  FunctionName=Lim_u16  EnableBusSupport=off  mask(Legacy Function){SFunctionSpec=uint16 y1 = Lim_u16(uint16 u1, uint16 u2, uint16 u3)}
      mask help:
      | This block allows you to call the legacy functions specified by the following Legacy Code Tool definition:
      | def.SFunctionName = 'Lim_u16';
      | def.OutputFcnSpec = 'uint16 y1 = Lim_u16(uint16 u1, uint16 u2, uint16 u3)';
      | def.HeaderFiles = {'NxtrMath.h', 'Std_Types.h', 'Platform_Types.h', 'Compiler.h', 'Compiler_Cfg.h'};
      | def.IncPaths = {'..\Nexteer_Utilities v3.0.0\SrcFiles'};
      settings: AttributesFormatString=%<Name>
      mask Help: <p>This block was generated automatically by the Legacy Code Tool. For detailed help on this tool, call<a href="matlab:legacy_code('help')"> legacy_code('help')</a>.</p>
      mask Display:
      | Xx = [-0.06, 0.06]*3;
      | Xy = [ 0, 0];
      | Yx = [ 0, 0];
      | Yy = [-0.14, 0.14]*3;
      | 
      | px = [-.06, -0.02, 0.02, 0.06]*3;
      | py = [-.1, -.1, .1, .1]*3;
      | plot(Xx+.5,Xy+.5, Yx+.5,Yy+.5, px+.5,py+.5)
      | port_label('input',1,'Inp')
      | port_label('input',2,'LoLim')
      | port_label('input',3,'HiLim')
      | port_label('output',1,'Outp')
  Out1 : Outport
  wires:
  Inp/1 -> Lim_u16/1
  LoLim/1 -> Lim_u16/2
  HiLim/1 -> Lim_u16/3
  Lim_u16/1 -> Out1/1

== system NxtrLim/LimDyn_u32/Lim_u32 ==
  Inp : Inport
  LoLim : Inport  Port=2
  HiLim : Inport  Port=3
  Lim_u32 : S-Function  FunctionName=Lim_u32  EnableBusSupport=off  mask(Legacy Function){SFunctionSpec=uint32 y1 = Lim_u32(uint32 u1, uint32 u2, uint32 u3)}
      mask help:
      | This block allows you to call the legacy functions specified by the following Legacy Code Tool definition:
      | def.SFunctionName = 'Lim_u32';
      | def.OutputFcnSpec = 'uint32 y1 = Lim_u32(uint32 u1, uint32 u2, uint32 u3)';
      | def.HeaderFiles = {'NxtrMath.h', 'Std_Types.h', 'Platform_Types.h', 'Compiler.h', 'Compiler_Cfg.h'};
      | def.IncPaths = {'..\Nexteer_Utilities v3.0.0\SrcFiles'};
      settings: AttributesFormatString=%<Name>
      mask Help: <p>This block was generated automatically by the Legacy Code Tool. For detailed help on this tool, call<a href="matlab:legacy_code('help')"> legacy_code('help')</a>.</p>
      mask Display:
      | Xx = [-0.06, 0.06]*3;
      | Xy = [ 0, 0];
      | Yx = [ 0, 0];
      | Yy = [-0.14, 0.14]*3;
      | 
      | px = [-.06, -0.02, 0.02, 0.06]*3;
      | py = [-.1, -.1, .1, .1]*3;
      | plot(Xx+.5,Xy+.5, Yx+.5,Yy+.5, px+.5,py+.5)
      | port_label('input',1,'Inp')
      | port_label('input',2,'LoLim')
      | port_label('input',3,'HiLim')
      | port_label('output',1,'Outp')
  Out1 : Outport
  wires:
  Lim_u32/1 -> Out1/1
  HiLim/1 -> Lim_u32/3
  LoLim/1 -> Lim_u32/2
  Inp/1 -> Lim_u32/1

== system NxtrLim/LimStat_s32/Lim_s32 ==
  Inp : Inport
  LoLim : Inport  Port=2
  HiLim : Inport  Port=3
  Lim_s32 : S-Function  FunctionName=Lim_s32  EnableBusSupport=off  mask(Legacy Function){SFunctionSpec=int32 y1 = Lim_s32( int32 u1,  int32 u2,  int32 u3)}
      mask help:
      | This block allows you to call the legacy functions specified by the following Legacy Code Tool definition:
      | def.SFunctionName = 'Lim_s32';
      | def.OutputFcnSpec = ' int32 y1 = Lim_s32( int32 u1,  int32 u2,  int32 u3)';
      | def.HeaderFiles = {'NxtrMath.h', 'Std_Types.h', 'Platform_Types.h', 'Compiler.h', 'Compiler_Cfg.h'};
      | def.IncPaths = {'..\Nexteer_Utilities v3.0.0\SrcFiles'};
      settings: AttributesFormatString=%<Name>
      mask Help: <p>This block was generated automatically by the Legacy Code Tool. For detailed help on this tool, call<a href="matlab:legacy_code('help')"> legacy_code('help')</a>.</p>
      mask Display:
      | Xx = [-0.06, 0.06]*3;
      | Xy = [ 0, 0];
      | Yx = [ 0, 0];
      | Yy = [-0.14, 0.14]*3;
      | 
      | px = [-.06, -0.02, 0.02, 0.06]*3;
      | py = [-.1, -.1, .1, .1]*3;
      | plot(Xx+.5,Xy+.5, Yx+.5,Yy+.5, px+.5,py+.5)
      | port_label('input',1,'Inp')
      | port_label('input',2,'LoLim')
      | port_label('input',3,'HiLim')
      | port_label('output',1,'Outp')
  Out1 : Outport
  wires:
  Lim_s32/1 -> Out1/1
  HiLim/1 -> Lim_s32/3
  LoLim/1 -> Lim_s32/2
  Inp/1 -> Lim_s32/1
